simulink model "GalvoDoku_ProfTroll"  (R2015a)
settings: Solver=ode45  StartTime=0.0  StopTime=10.0  RelTol=1e-3
values from neighbouring files (symbols this model uses):
  FS = 2.0E-6    [dataDict_galvoSystemParams.sldd]    (also in ddict.mat = 2e-06; modelInitScript.m = 2e-06)
  JR = 7.3E-9    [dataDict_galvoLSK040EF.sldd]    (also in dataDict_galvoMod6860.sldd = 6.0E-8
  KEL = 0.015    [dataDict_galvoLSK040EF.sldd]    (also in dataDict_galvoMod6860.sldd = 0.0093
  KEMF = 0.007    [dataDict_galvoLSK040EF.sldd]    (also in dataDict_galvoMod6860.sldd = 0.00974
  KFR = 4.0E-6    [dataDict_galvoLSK040EF.sldd]    (also in dataDict_galvoMod6860.sldd = 1.0E-10
  KPD : value not decoded    [dataDict_galvoSystemParams.sldd]
  KTB = 0.047    [dataDict_galvoLSK040EF.sldd]    (also in dataDict_galvoMod6860.sldd = 1.0E-9
  L = 0.0018    [dataDict_galvoLSK040EF.sldd]    (also in dataDict_galvoMod6860.sldd = 0.00016
  RL = 2.3    [dataDict_galvoLSK040EF.sldd]    (also in dataDict_galvoMod6860.sldd = 1.5
  Rsh = 0.075    [dataDict_galvoSystemParams.sldd]    (also in modelInitScript.m = str2num(p.Rsh.v))
undefined symbols (not defined in the file or in its folder): BF, KBM, KME, KMT, Lc, Rc
libraries: simulink x1
settings Model: Creator=mainster  LastModifiedBy=mainster
settings DebuggingCC: UnderspecifiedInitializationDetection=Classic  MergeDetectMultiDrivingBlocksExec=none  SolverPrmCheckMsg=warning  StateNameClashWarn=warning

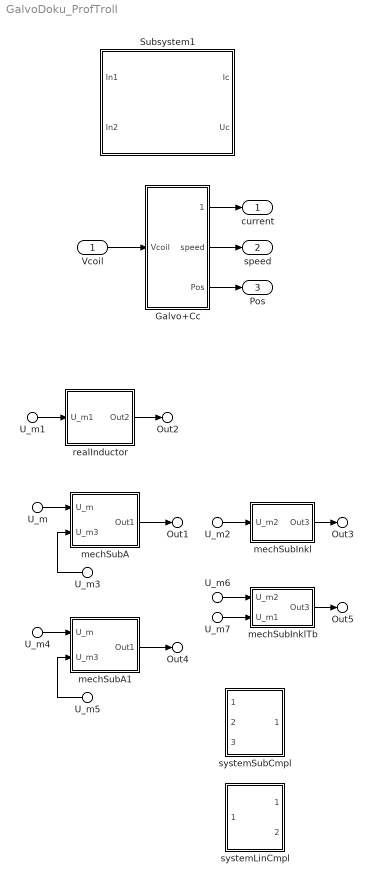
== system GalvoDoku_ProfTroll ==
  Vcoil : Inport
  U_m : Inport  Port=2
  U_m2 : Inport  Port=3
  U_m3 : Inport  Port=4
  U_m1 : Inport  Port=5
  U_m4 : Inport  Port=6
  U_m5 : Inport  Port=7
  U_m6 : Inport  Port=8
  U_m7 : Inport  Port=9
  Galvo+Cc : Subsystem
  Subsystem1 : Subsystem
      mask Display: text(.05,.05,['{\fontsize{13}\it\bfCurrent comp}'],'horizontalAlignment','left','verticalAlignment','bottom','texmode','on')
  mechSubA : Subsystem
  mechSubA1 : Subsystem
  mechSubInkl : Subsystem
  mechSubInklTb : Subsystem
  realInductor : Subsystem
      settings: AttributesFormatString=%<BlockType>
  systemLinCmpl : Subsystem
  systemSubCmpl : Subsystem
  current : Outport
  speed : Outport  Port=2
  Pos : Outport  Port=3
  Out1 : Outport  Port=4
  Out3 : Outport  Port=5
  Out2 : Outport  Port=6
  Out4 : Outport  Port=7
  Out5 : Outport  Port=8
  wires:
  Vcoil/1 -> Galvo+Cc/1(Vcoil)
  Galvo+Cc/1(current) -> current/1
  Galvo+Cc/2(speed) -> speed/1
  Galvo+Cc/3(Pos) -> Pos/1
  U_m1/1 -> realInductor/1(U_m1)
  realInductor/1(Out2) -> Out2/1
  U_m2/1 -> mechSubInkl/1(U_m2)
  mechSubInkl/1(Out3) -> Out3/1
  U_m/1 -> mechSubA/1(U_m)
  U_m3/1 -> mechSubA/2(U_m3)
  mechSubA/1(Out1) -> Out1/1
  U_m4/1 -> mechSubA1/1(U_m)
  U_m5/1 -> mechSubA1/2(U_m3)
  mechSubA1/1(Out1) -> Out4/1
  U_m6/1 -> mechSubInklTb/1(U_m2)
  mechSubInklTb/1(Out3) -> Out5/1
  U_m7/1 -> mechSubInklTb/2(U_m1)

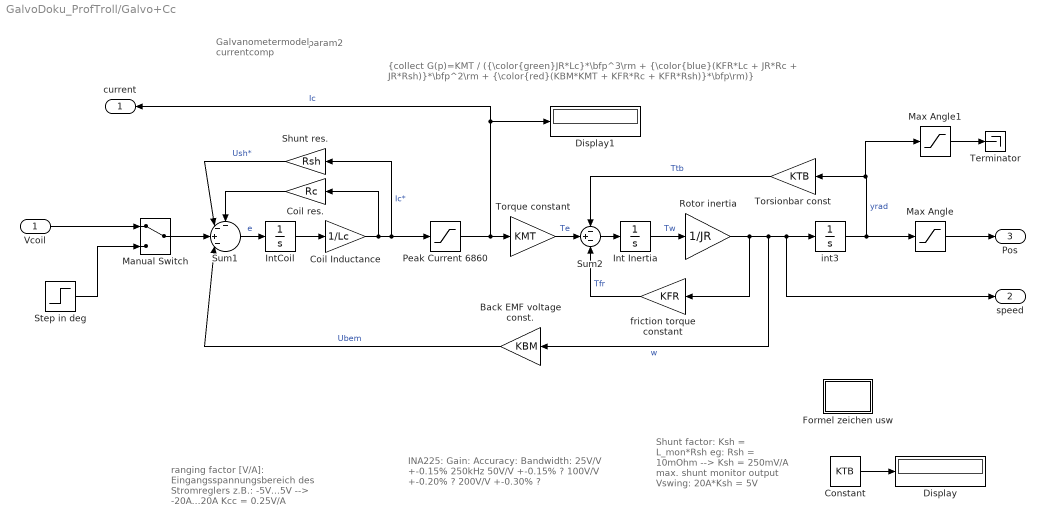
== system GalvoDoku_ProfTroll/Galvo+Cc ==
  note: {collect G(p)=KMT / ({\color{green}JR*Lc}*\bfp^3\rm + {\color{blue}(KFR*Lc + JR*Rc + JR*Rsh)}*\bfp^2\rm + {\color{red}(KBM*KMT + KFR*Rc + KFR*Rsh)}*\bfp\rm)}
  note: param2
  note: Galvanometermodel
      | currentcomp
  note: ranging factor [V/A]:
      | Eingangsspannungsbereich des
      | Stromreglers z.B.:
      | -5V...5V --> -20A...20A
      | Kcc = 0.25V/A
  note: Shunt factor:
      | Ksh = L_mon*Rsh
      |
      | eg: Rsh = 10mOhm
      |
      | --> Ksh = 250mV/A
      | max. shunt monitor
      | output Vswing:
      | 20A*Ksh = 5V
  note: INA225:
      | Gain:		Accuracy:		Bandwidth:
      | 25V/V		+-0.15%		250kHz
      | 50V/V		+-0.15%		?
      | 100V/V	+-0.20%		?
      | 200V/V	+-0.30%		?
  Vcoil : Inport
  Back EMF voltage const. : Gain  Gain=KBM
  Coil Inductance : Gain  Gain=1/Lc
  Coil res. : Gain  Gain=Rc
  Constant : Constant  Value=KTB  SampleTime=-1
  Display : Display
  Display1 : Display
  Formel zeichen usw : Subsystem
  Int Inertia : Integrator
  IntCoil : Integrator
  Manual Switch : ManualSwitch
  Max Angle : Saturate  UpperLimit=20*pi/180  LowerLimit=-20*pi/180
      settings: AttributesFormatString=Max=%<UpperLimit>\nMin=%<LowerLimit>
  Max Angle1 : Saturate  UpperLimit=20  LowerLimit=-20
      settings: AttributesFormatString=Max=%<UpperLimit>\nMin=%<LowerLimit>
  Peak Current 6860 : Saturate  UpperLimit=30  LowerLimit=-30
      settings: AttributesFormatString=+-%<UpperLimit>A
  Rotor inertia : Gain  Gain=1/JR
  Shunt res. : Gain  Gain=Rsh
  Step in deg : Step  Time=1e-3  SampleTime=FS  ZeroCross=off
      settings: AttributesFormatString=Ampl.: %<After>\ntime:%<Time>
  Sum1 : Sum  Inputs=--+-|
  Sum2 : Sum  Inputs=-+-
  Terminator : Terminator
  Torque constant : Gain  Gain=KMT
  Torsionbar const : Gain  Gain=KTB
  friction torque constant : Gain  Gain=KFR
  int3 : Integrator
  current : Outport
  speed : Outport  Port=2
  Pos : Outport  Port=3
  wires:
  Shunt res./1 -> Sum1/2  "Ush*"
  IntCoil/1 -> Coil Inductance/1
  Torsionbar const/1 -> Sum2/1  "Ttb"
  Torque constant/1 -> Sum2/2  "Te"
  Int Inertia/1 -> Rotor inertia/1  "Tw"
  Max Angle/1 -> Pos/1
  Peak Current 6860/1 -> current/1, Display1/1, Torque constant/1  "Ic"
  Sum1/1 -> IntCoil/1  "e"
  Constant/1 -> Display/1
  Rotor inertia/1 -> friction torque constant/1, speed/1, int3/1, Back EMF voltage const./1  "w"
  Manual Switch/1 -> Sum1/3
  Sum2/1 -> Int Inertia/1
  Coil res./1 -> Sum1/1
  Vcoil/1 -> Manual Switch/1
  Back EMF voltage const./1 -> Sum1/4  "Ubem"
  friction torque constant/1 -> Sum2/3  "Tfr"
  int3/1 -> Max Angle/1, Max Angle1/1, Torsionbar const/1  "yrad"
  Coil Inductance/1 -> Coil res./1, Shunt res./1, Peak Current 6860/1  "Ic*"
  Step in deg/1 -> Manual Switch/2
  Max Angle1/1 -> Terminator/1

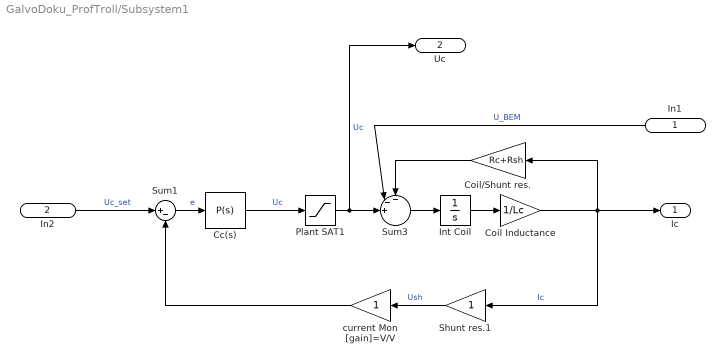
== system GalvoDoku_ProfTroll/Subsystem1 ==
  In1 : Inport
  In2 : Inport  Port=2
  Cc(s) : simulink/Continuous/PID Controller  Controller=P  TimeDomain=Continuous-time  SampleTime=-1  IntegratorMethod=Forward Euler  FilterMethod=Forward Euler  Form=Ideal  UseFilter=on  ControllerParametersSource=internal  P=18.7463154861029  I=14078.2261040339  D=0  N=100  InitialConditionSource=internal  InitialConditionForIntegrator=0  InitialConditionForFilter=0  ExternalReset=none  LimitOutput=off  UpperSaturationLimit=inf  LowerSaturationLimit=-inf  LinearizeAsGain=on  AntiWindupMode=none  Kb=1  TrackingMode=off  Kt=1  PParamMin=[]  PParamMax=[]  IParamMin=[]  IParamMax=[]  DParamMin=[]  DParamMax=[]  NParamMin=[]  NParamMax=[]  KbParamMin=[]  KbParamMax=[]  KtParamMin=[]  KtParamMax=[]  POutMin=[]  POutMax=[]  IOutMin=[]  IOutMax=[]  DOutMin=[]  DOutMax=[]  NOutMin=[]  NOutMax=[]  KbOutMin=[]  KbOutMax=[]  KtOutMin=[]  KtOutMax=[]  IntegratorOutMin=[]  IntegratorOutMax=[]  FilterOutMin=[]  FilterOutMax=[]  SumOutMin=[]  SumOutMax=[]  SumI1OutMin=[]  SumI1OutMax=[]  SumI2OutMin=[]  SumI2OutMax=[]  SumI3OutMin=[]  SumI3OutMax=[]  SumDOutMin=[]  SumDOutMax=[]  SaturationOutMin=[]  SaturationOutMax=[]  IntegratorContinuousStateAttributes=''  IntegratorStateMustResolveToSignalObject=off  IntegratorRTWStateStorageClass=Auto  FilterContinuousStateAttributes=''  FilterStateMustResolveToSignalObject=off  FilterRTWStateStorageClass=Auto  DifferentiatorICPrevScaledInput=0  DifferentiatorOutMin=[]  DifferentiatorOutMax=[]
  Coil Inductance : Gain  Gain=1/Lc
  Coil/Shunt res. : Gain  Gain=Rc+Rsh
  Int Coil : Integrator
  Plant SAT1 : Saturate  UpperLimit=30  LowerLimit=-30
      settings: AttributesFormatString=U_lim=+-%<UpperLimit>V
  Shunt res.1 : Gain
  Sum1 : Sum  Inputs=|+-
  Sum3 : Sum  Inputs=--+||
  current Mon [gain]=V/V : Gain
  Ic : Outport
  Uc : Outport  Port=2
  wires:
  Sum1/1 -> Cc(s)/1  "e"
  Coil Inductance/1 -> Ic/1, Shunt res.1/1, Coil/Shunt res./1  "Ic"
  Coil/Shunt res./1 -> Sum3/1
  Sum3/1 -> Int Coil/1
  Int Coil/1 -> Coil Inductance/1
  Cc(s)/1 -> Plant SAT1/1  "Uc"
  Shunt res.1/1 -> current Mon [gain]=V/V/1  "Ush"
  current Mon [gain]=V/V/1 -> Sum1/2
  Plant SAT1/1 -> Uc/1, Sum3/3  "Uc"
  In1/1 -> Sum3/2  "U_BEM"
  In2/1 -> Sum1/1  "Uc_set"

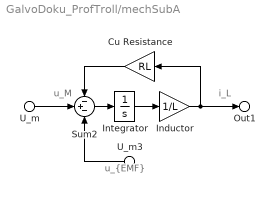
== system GalvoDoku_ProfTroll/mechSubA ==
  note: u_M
  note: i_L
  note: u_{EMF}
  U_m : Inport
  U_m3 : Inport  Port=2
  Cu Resistance : Gain  Gain=RL
  Inductor : Gain  Gain=1/L
  Integrator : Integrator
  Sum2 : Sum  Inputs=-+-
  Out1 : Outport
  wires:
  Sum2/1 -> Integrator/1
  Cu Resistance/1 -> Sum2/1
  Integrator/1 -> Inductor/1
  U_m3/1 -> Sum2/3
  U_m/1 -> Sum2/2
  Inductor/1 -> Out1/1, Cu Resistance/1

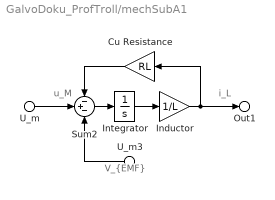
== system GalvoDoku_ProfTroll/mechSubA1 ==
  note: u_M
  note: i_L
  note: V_{EMF}
  U_m : Inport
  U_m3 : Inport  Port=2
  Cu Resistance : Gain  Gain=RL
  Inductor : Gain  Gain=1/L
  Integrator : Integrator
  Sum2 : Sum  Inputs=-+-
  Out1 : Outport
  wires:
  Sum2/1 -> Integrator/1
  Cu Resistance/1 -> Sum2/1
  Integrator/1 -> Inductor/1
  U_m3/1 -> Sum2/3
  U_m/1 -> Sum2/2
  Inductor/1 -> Out1/1, Cu Resistance/1

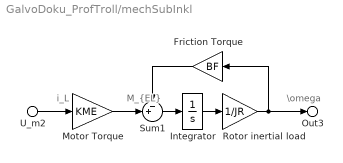
== system GalvoDoku_ProfTroll/mechSubInkl ==
  note: M_{EL}
  note: \omega
  note: i_L
  U_m2 : Inport
  Friction Torque : Gain  Gain=BF
  Integrator : Integrator
  Motor Torque : Gain  Gain=KME
  Rotor inertial load : Gain  Gain=1/JR
  Sum1 : Sum  Inputs=-+|
  Out3 : Outport
  wires:
  Sum1/1 -> Integrator/1
  Integrator/1 -> Rotor inertial load/1
  Friction Torque/1 -> Sum1/1
  U_m2/1 -> Motor Torque/1
  Motor Torque/1 -> Sum1/2
  Rotor inertial load/1 -> Out3/1, Friction Torque/1

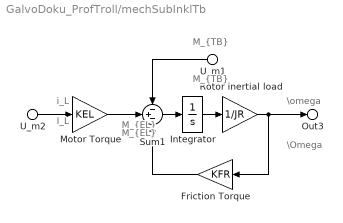
== system GalvoDoku_ProfTroll/mechSubInklTb ==
  note: M_{EL}
  note: \omega
  note: i_L
  note: I_L
  note: M_{EL}
  note: \Omega
  note: M_{TB}
  note: M_{TB}
  U_m2 : Inport
  U_m1 : Inport  Port=2
  Friction Torque : Gain  Gain=KFR
  Integrator : Integrator
  Motor Torque : Gain  Gain=KEL
  Rotor inertial load : Gain  Gain=1/JR
  Sum1 : Sum  Inputs=-+-
  Out3 : Outport
  wires:
  Sum1/1 -> Integrator/1
  Integrator/1 -> Rotor inertial load/1
  Friction Torque/1 -> Sum1/3
  U_m2/1 -> Motor Torque/1
  Motor Torque/1 -> Sum1/2
  Rotor inertial load/1 -> Out3/1, Friction Torque/1
  U_m1/1 -> Sum1/1

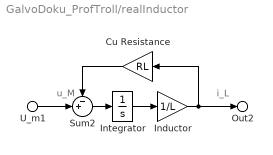
== system GalvoDoku_ProfTroll/realInductor ==
  note: u_M
  note: i_L
  U_m1 : Inport
  Cu Resistance : Gain  Gain=RL
  Inductor : Gain  Gain=1/L
  Integrator : Integrator
  Sum2 : Sum  Inputs=-+|
  Out2 : Outport
  wires:
  U_m1/1 -> Sum2/2
  Sum2/1 -> Integrator/1
  Inductor/1 -> Out2/1, Cu Resistance/1
  Integrator/1 -> Inductor/1
  Cu Resistance/1 -> Sum2/1

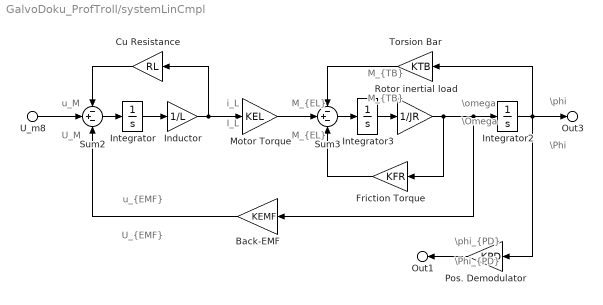
== system GalvoDoku_ProfTroll/systemLinCmpl ==
  note: \Phi
  note: \phi
  note: u_M
  note: M_{EL}
  note: \omega
  note: i_L
  note: I_L
  note: M_{EL}
  note: \Omega
  note: M_{TB}
  note: M_{TB}
  note: U_M
  note: u_{EMF}
  note: U_{EMF}
  note: \Phi_{PD}
  note: \phi_{PD}
  U_m8 : Inport
  Back-EMF : Gain  Gain=KEMF
  Cu Resistance : Gain  Gain=RL
  Friction Torque : Gain  Gain=KFR
  Inductor : Gain  Gain=1/L
  Integrator : Integrator
  Integrator2 : Integrator
  Integrator3 : Integrator
  Motor Torque : Gain  Gain=KEL
  Pos. Demodulator : Gain  Gain=KPD
  Rotor inertial load : Gain  Gain=1/JR
  Sum2 : Sum  Inputs=-+-
  Sum3 : Sum  Inputs=-+-
  Torsion Bar : Gain  Gain=KTB
  Out3 : Outport
  Out1 : Outport  Port=2
  wires:
  Back-EMF/1 -> Sum2/3
  Sum2/1 -> Integrator/1
  Cu Resistance/1 -> Sum2/1
  U_m8/1 -> Sum2/2
  Integrator/1 -> Inductor/1
  Inductor/1 -> Motor Torque/1, Cu Resistance/1
  Motor Torque/1 -> Sum3/2
  Integrator2/1 -> Pos. Demodulator/1, Torsion Bar/1, Out3/1
  Sum3/1 -> Integrator3/1
  Integrator3/1 -> Rotor inertial load/1
  Friction Torque/1 -> Sum3/3
  Torsion Bar/1 -> Sum3/1
  Rotor inertial load/1 -> Back-EMF/1, Integrator2/1, Friction Torque/1
  Pos. Demodulator/1 -> Out1/1

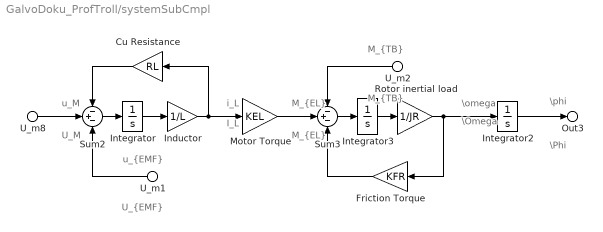
== system GalvoDoku_ProfTroll/systemSubCmpl ==
  note: \Phi
  note: \phi
  note: u_M
  note: u_{EMF}
  note: M_{EL}
  note: \omega
  note: i_L
  note: I_L
  note: M_{EL}
  note: \Omega
  note: M_{TB}
  note: M_{TB}
  note: U_M
  note: U_{EMF}
  U_m8 : Inport
  U_m1 : Inport  Port=2
  U_m2 : Inport  Port=3
  Cu Resistance : Gain  Gain=RL
  Friction Torque : Gain  Gain=KFR
  Inductor : Gain  Gain=1/L
  Integrator : Integrator
  Integrator2 : Integrator
  Integrator3 : Integrator
  Motor Torque : Gain  Gain=KEL
  Rotor inertial load : Gain  Gain=1/JR
  Sum2 : Sum  Inputs=-+-
  Sum3 : Sum  Inputs=-+-
  Out3 : Outport
  wires:
  U_m1/1 -> Sum2/3
  Sum2/1 -> Integrator/1
  Cu Resistance/1 -> Sum2/1
  U_m8/1 -> Sum2/2
  Integrator/1 -> Inductor/1
  Inductor/1 -> Motor Torque/1, Cu Resistance/1
  Motor Torque/1 -> Sum3/2
  Integrator2/1 -> Out3/1
  Sum3/1 -> Integrator3/1
  Integrator3/1 -> Rotor inertial load/1
  Friction Torque/1 -> Sum3/3
  U_m2/1 -> Sum3/1
  Rotor inertial load/1 -> Integrator2/1, Friction Torque/1

== system GalvoDoku_ProfTroll/Galvo+Cc/Formel zeichen usw ==
  note: Te: 		electrical torque, gen. by coils		[Nm]
      |  Ic: 			coil current							[A]
      |  Tfr:		rotor dynamic friction torque 		[Nm]
      |  Trb:		torsion bar torque					[Nm]
      |  Tw:		angular momentum				[Nm*s]
      |  w:			angular velocity 					[rad/s]
      |  yrad:		angular position 					[rad]
      |  ydeg:		angular position 					[°]
      |  Ucci:		current controller input				[V]
      |  Ucco:		current controller output			[V]
      |  Ush:		shunt voltage						[V]
  note: balance of force: 	Te=Ttb+Tfr
      | 					Te - (Ttb+Tfr)=0  ->  no movement
      |
      |  integrate( 1 Nm )dt = 1 Nm*s
      |  (Nm*s)(kg*m²)⁻¹ = (N*s/kg)*m⁻¹ = m/(s*m) = rad
  note: L_{c  }	coil inductance 							[H]
      |  R_{c  }	coil resistance							[\Omega]
      |  R_{SH }	current shunt resistance				[\Omega]
      |  J_{R  }	rotor inertia 							[kg*m²]
      |  \color{red}K_{TB }	torsion bar torque const. 			[Nm/rad]
      |  \color{black}K_{BM }	back EMF const.							[V*s/rad]
      |  K_{FR }	rotor dyn. friction torque const.	[Nm*s/rad]
      |  K_{MT }	el. magnetic torque const.			[Nm/A]
